simulink model "sampleModel1"  (R2021a)
settings: Solver=VariableStepAuto  StartTime=0.0  StopTime=50  RelTol=1e-3
undefined symbols (not defined in the file): DiscIntNeverNeededParam, magnitude, Newton, Raphson
libraries: simulink x92, pid_lib x10
(part 5 of 5)

== system sampleModel1/cfblk91/cfblk18/cfblk15/cfblk12 ==
  cfblk1 : Inport
  cfblk15 : Inport  Port=2
  cfblk16 : Inport  Port=3
  Action Port : ActionPort  ActionPortLabel=else
  cfblk10 : Constant  Value=[-246777843.934526]  SampleTime=1
  cfblk11 : Constant  Value=[569704854.566047]  SampleTime=1
  cfblk12 : Constant  Value=[627953853.641868]  SampleTime=1
  cfblk13 : Constant  Value=[-141522913.770345]  SampleTime=1
  cfblk14 : Constant  Value=[193294208.890492]  SampleTime=1
  cfblk3 : pid_lib/PID Controller  Controller=PID  Form=Parallel  TimeDomain=Discrete-time  UseExternalTs=off  SampleTime=-1  IntegratorMethod=Forward Euler  FilterMethod=Forward Euler  ControllerParametersSource=internal  P=1  I=1  D=0  UseFilter=on  N=100  TunerSelectOption=Transfer Function Based (PID Tuner App)  InitialConditionSource=internal  InitialConditionForIntegrator=0  InitialConditionForFilter=0  DifferentiatorICPrevScaledInput=0  ExternalReset=none  TrackingMode=off  Kt=1  LimitOutput=off  SatLimitsSource=internal  UpperSaturationLimit=inf  LowerSaturationLimit=-inf  LinearizeAsGain=off  AntiWindupMode=none  Kb=1  POutMin=[]  POutMax=[]  IOutMin=[]  IOutMax=[]  DOutMin=[]  DOutMax=[]  NOutMin=[]  NOutMax=[]  SumOutMin=[]  SumOutMax=[]  SaturationOutMin=[]  SaturationOutMax=[]  PParamMin=[]  PParamMax=[]  IParamMin=[]  IParamMax=[]  DParamMin=[]  DParamMax=[]  NParamMin=[]  NParamMax=[]  KbParamMin=[]  KbParamMax=[]  KtParamMin=[]  KtParamMax=[]  KbOutMin=[]  KbOutMax=[]  KtOutMin=[]  KtOutMax=[]  IntegratorOutMin=[]  IntegratorOutMax=[]  FilterOutMin=[]  FilterOutMax=[]  SumI1OutMin=[]  SumI1OutMax=[]  SumI2OutMin=[]  SumI2OutMax=[]  SumI3OutMin=[]  SumI3OutMax=[]  SumI4OutMin=[]  SumI4OutMax=[]  SumDOutMin=[]  SumDOutMax=[]  DifferentiatorOutMin=[]  DifferentiatorOutMax=[]  FilterDiffOutCoefMin=[]  FilterDiffOutCoefMax=[]  ReciprocalOutMin=[]  ReciprocalOutMax=[]  SumDenOutMin=[]  SumDenOutMax=[]  SumNumOutMin=[]  SumNumOutMax=[]  DivideOutMin=[]  DivideOutMax=[]  UdiffTsProdOutMin=[]  UdiffTsProdOutMax=[]  NTsProdOutMin=[]  NTsProdOutMax=[]  UintegralTsProdOutMin=[]  UintegralTsProdOutMax=[]  UngainTsProdOutMin=[]  UngainTsProdOutMax=[]  IntegratorContinuousStateAttributes=''  IntegratorStateMustResolveToSignalObject=off  IntegratorRTWStateStorageClass=Auto  FilterContinuousStateAttributes=''  FilterStateMustResolveToSignalObject=off  FilterRTWStateStorageClass=Auto  ParallelPVariant=InternalParameters  IdealPVariant=Disabled  IVariant=InternalParameters  DVariant=InternalParameters  IntegratorVariant=Discrete  SatVariant=Disabled  AWVariant=Passthrough  PCopyVariant=Disabled  TRVariant=Disabled  FdbkBlocksVariant=Forward  IdealPFdbkVariant=Disabled  SatFdbkVariant=Disabled  DerivativeFilterVariant=ForwardEulerFilter  NVariant=InternalParameters  NCopyVariant=Disabled  FilterICVariant=InternalICsFilter  IntegratorICVariant=InternalICs  ExternalResetVariant=Disabled  TRSumVariant=Passthrough  SumFdbkVariant=Disabled  SumVariant=Sum_PID  TsampFilterVariant=InternalTs  TsampNgainVariant=Passthrough  TsampIntegralVariant=Passthrough  ExternalSaturationOutDataTypeStr=Inherit: Same as second input
  cfblk4 : DiscreteZeroPole  Poles=[0 0.5]  Gain=1  SampleTime=-1
  cfblk5 : Gain  Gain=[-57796269.968503]
  cfblk6 : Product  Inputs=**
  cfblk7 : Product  Inputs=**
  cfblk8 : Sum  Inputs=|++
  cfblk9 : Constant  Value=[688974792.966896]  SampleTime=1
  cfblk2 : Outport
  cfblk17 : Outport  Port=2
  wires:
  cfblk8/1 -> cfblk7/1
  cfblk16/1 -> cfblk7/2
  cfblk10/1 -> cfblk5/1
  cfblk1/1 -> cfblk3/1
  cfblk4/1 -> cfblk2/1
  cfblk3/1 -> cfblk6/1
  cfblk12/1 -> cfblk17/1
  cfblk5/1 -> cfblk4/1
  cfblk11/1 -> cfblk6/2
  cfblk6/1 -> cfblk8/1
  cfblk9/1 -> cfblk8/2

== system sampleModel1/cfblk91/cfblk18/cfblk15/cfblk9 ==
  cfblk1 : Inport
  cfblk7 : Inport  Port=2
  Action Port : ActionPort  ActionPortLabel=if(u1 >= 0)
  cfblk3 : DiscreteIntegrator  SampleTime=-1  ICPrevOutput=DiscIntNeverNeededParam  ICPrevScaledInput=DiscIntNeverNeededParam
  cfblk4 : Squeeze
  cfblk5 : Constant  Value=[717518068.143608]  SampleTime=1
  cfblk6 : Constant  Value=[-364333892.547543]  SampleTime=1
  cfblk2 : Outport
  wires:
  cfblk1/1 -> cfblk4/1
  cfblk4/1 -> cfblk2/1
  cfblk7/1 -> cfblk3/1

== system sampleModel1/cfblk92/cfblk17/cfblk11/cfblk14 ==
  cfblk1 : Inport
  cfblk10 : Inport  Port=2
  cfblk11 : Inport  Port=3
  cfblk12 : Inport  Port=4
  cfblk13 : Inport  Port=5
  cfblk14 : Inport  Port=6
  Action Port : ActionPort  ActionPortLabel=if(u1 >= 0)
  cfblk3 : Gain  Gain=[-441921625.450770]
  cfblk4 : PermuteDimensions
  cfblk5 : Sqrt  SaturateOnIntegerOverflow=on
  cfblk6 : simulink/Math Operations/MinMax Running Resettable  Function=min  vinit=0.0
  cfblk7 : PermuteDimensions
  cfblk8 : Constant  Value=[350750636.833189]  SampleTime=1
  cfblk9 : Constant  Value=[817051797.696749]  SampleTime=1
  cfblk2 : Outport
  cfblk15 : Outport  Port=2
  wires:
  cfblk11/1 -> cfblk3/1
  cfblk3/1 -> cfblk2/1
  cfblk5/1 -> cfblk4/1
  cfblk1/1 -> cfblk7/1
  cfblk12/1 -> cfblk15/1
  cfblk9/1 -> cfblk6/1
  cfblk14/1 -> cfblk6/2
  cfblk6/1 -> cfblk5/1

== system sampleModel1/cfblk92/cfblk17/cfblk11/cfblk15 ==
  cfblk1 : Inport
  Action Port : ActionPort  ActionPortLabel=else
  cfblk10 : Trigonometry
  cfblk11 : Constant  Value=[197257053.266469]  SampleTime=1
  cfblk12 : Constant  Value=[592490701.451690]  SampleTime=1
  cfblk13 : Constant  Value=[-859572952.026083]  SampleTime=1
  cfblk14 : Constant  Value=[-727985222.759821]  SampleTime=1
  cfblk18 : Delay
  cfblk19 : Delay
  cfblk3 : DiscreteIntegrator  SampleTime=-1  ICPrevOutput=DiscIntNeverNeededParam  ICPrevScaledInput=DiscIntNeverNeededParam
  cfblk4 : Delay
  cfblk5 : Squeeze
  cfblk6 : Math  SaturateOnIntegerOverflow=on
  cfblk7 : Sum  Inputs=+-
  cfblk8 : DotProduct  InputSameDT=on  OutDataTypeStr=Inherit: Inherit via internal rule
  cfblk9 : Sum  Inputs=+-
  cfblk2 : Outport
  cfblk15 : Outport  Port=2
  cfblk16 : Outport  Port=3
  cfblk17 : Outport  Port=4
  wires:
  cfblk5/1 -> cfblk6/1, cfblk18/1
  cfblk3/1 -> cfblk5/1
  cfblk11/1 -> cfblk16/1
  cfblk9/1 -> cfblk10/1
  cfblk6/1 -> cfblk8/1, cfblk7/2
  cfblk1/1 -> cfblk9/1
  cfblk7/1 -> cfblk4/1
  cfblk14/1 -> cfblk17/1
  cfblk10/1 -> cfblk2/1
  cfblk8/1 -> cfblk9/2
  cfblk12/1 -> cfblk15/1
  cfblk13/1 -> cfblk8/2
  cfblk18/1 -> cfblk3/1
  cfblk4/1 -> cfblk19/1
  cfblk19/1 -> cfblk7/1

== system sampleModel1/cfblk92/cfblk17/cfblk11/cfblk7 ==
  cfblk1 : Inport
  cfblk10 : Constant  Value=[697193350.959098]  SampleTime=1
  cfblk11 : Constant  Value=[-67596332.418728]  SampleTime=1
  cfblk12 : Constant  Value=[260410249.999499]  SampleTime=1
  cfblk3 : DiscreteFilter
  cfblk4 : simulink/Discrete/Difference  ICPrevInput=0.0  OutMin=[]  OutMax=[]  OutDataTypeStr=Inherit: Inherit via back propagation  OutDataType=fixdt(1, 16)  OutScaling=2^-10  DoSatur=off
  cfblk5 : simulink/Math Operations/Slider Gain  gain=1  low=0  high=2
  cfblk6 : Gain  Gain=[566531874.808073]
  cfblk7 : Sum  Inputs=|++
  cfblk8 : simulink/Math Operations/MinMax Running Resettable  Function=min  vinit=0.0
  cfblk9 : Constant  Value=[-772138722.643148]  SampleTime=1
  cfblk2 : Outport
  cfblk13 : Outport  Port=2
  cfblk14 : Outport  Port=3
  wires:
  cfblk9/1 -> cfblk7/1
  cfblk6/1 -> cfblk7/2
  cfblk7/1 -> cfblk2/1
  cfblk1/1 -> cfblk5/1
  cfblk8/1 -> cfblk6/1
  cfblk11/1 -> cfblk8/1
  cfblk12/1 -> cfblk13/1
  cfblk4/1 -> cfblk3/1
  cfblk10/1 -> cfblk8/2
  cfblk3/1 -> cfblk14/1
  cfblk5/1 -> cfblk4/1

== system sampleModel1/cfblk92/cfblk17/cfblk11/cfblk8 ==
  cfblk1 : Inport
  cfblk12 : Inport  Port=2
  cfblk13 : Inport  Port=3
  cfblk14 : Inport  Port=4
  cfblk10 : Constant  Value=[633710347.547700]  SampleTime=1
  cfblk11 : Constant  Value=[388701121.244883]  SampleTime=1
  cfblk3 : simulink/Discrete/Difference  ICPrevInput=0.0  OutMin=[]  OutMax=[]  OutDataTypeStr=Inherit: Inherit via back propagation  OutDataType=fixdt(1, 16)  OutScaling=2^-10  DoSatur=off
  cfblk4 : Sum  Inputs=|++
  cfblk5 : Abs
  cfblk6 : Gain  Gain=[852588536.395900]
  cfblk7 : Constant  Value=[-863639126.345931]  SampleTime=1
  cfblk8 : Constant  Value=[274302445.050449]  SampleTime=1
  cfblk9 : Constant  Value=[729244025.067106]  SampleTime=1
  cfblk2 : Outport
  cfblk15 : Outport  Port=2
  wires:
  cfblk11/1 -> cfblk5/1
  cfblk7/1 -> cfblk15/1
  cfblk1/1 -> cfblk2/1
  cfblk13/1 -> cfblk4/1
  cfblk5/1 -> cfblk6/1
  cfblk9/1 -> cfblk4/2
  cfblk4/1 -> cfblk3/1

== system sampleModel1/cfblk92/cfblk18/cfblk10/cfblk11 ==
  cfblk1 : Inport
  cfblk6 : Inport  Port=2
  cfblk7 : Inport  Port=3
  cfblk3 : DiscreteFilter
  cfblk4 : Reshape
  cfblk5 : Constant  Value=[-313988376.059350]  SampleTime=1
  cfblk2 : Outport
  cfblk8 : Outport  Port=2
  wires:
  cfblk6/1 -> cfblk8/1
  cfblk4/1 -> cfblk2/1
  cfblk1/1 -> cfblk3/1
  cfblk5/1 -> cfblk4/1

== system sampleModel1/cfblk92/cfblk18/cfblk6/cfblk11 ==
  cfblk1 : Inport
  cfblk11 : Inport  Port=2
  Action Port : ActionPort  ActionPortLabel=if(u1 >= 0)
  cfblk10 : Constant  Value=[-988693863.746309]  SampleTime=1
  cfblk3 : simulink/Math Operations/MinMax Running Resettable  Function=min  vinit=0.0
  cfblk4 : Product  Inputs=**
  cfblk5 : Product  Inputs=**
  cfblk6 : Product
  cfblk7 : Constant  Value=[-726696956.202840]  SampleTime=1
  cfblk8 : Constant  Value=[-600331750.665850]  SampleTime=1
  cfblk9 : Constant  Value=[86089967.308776]  SampleTime=1
  cfblk2 : Outport
  cfblk12 : Outport  Port=2
  wires:
  cfblk5/1 -> cfblk6/1
  cfblk8/1 -> cfblk2/1
  cfblk10/1 -> cfblk3/1, cfblk4/2
  cfblk3/1 -> cfblk5/1
  cfblk9/1 -> cfblk12/1
  cfblk1/1 -> cfblk6/2
  cfblk7/1 -> cfblk3/2
  cfblk11/1 -> cfblk5/2
  cfblk6/1 -> cfblk4/1

== system sampleModel1/cfblk92/cfblk18/cfblk6/cfblk12 ==
  cfblk1 : Inport
  cfblk10 : Inport  Port=2
  cfblk11 : Inport  Port=3
  Action Port : ActionPort  ActionPortLabel=else
  cfblk3 : simulink/Discrete/Difference  ICPrevInput=0.0  OutMin=[]  OutMax=[]  OutDataTypeStr=Inherit: Inherit via back propagation  OutDataType=fixdt(1, 16)  OutScaling=2^-10  DoSatur=off
  cfblk4 : DiscreteFir
  cfblk5 : Abs
  cfblk6 : simulink/Math Operations/MinMax Running Resettable  Function=min  vinit=0.0
  cfblk7 : Constant  Value=[82707866.615409]  SampleTime=1
  cfblk8 : Constant  Value=[-403001105.881521]  SampleTime=1
  cfblk9 : Constant  Value=[718960214.413579]  SampleTime=1
  cfblk2 : Outport
  cfblk12 : Outport  Port=2
  cfblk13 : Outport  Port=3
  cfblk14 : Outport  Port=4
  wires:
  cfblk7/1 -> cfblk3/1
  cfblk5/1 -> cfblk13/1
  cfblk9/1 -> cfblk12/1
  cfblk6/1 -> cfblk5/1
  cfblk1/1 -> cfblk14/1
  cfblk8/1 -> cfblk2/1
  cfblk11/1 -> cfblk6/1
  cfblk3/1 -> cfblk4/1
  cfblk4/1 -> cfblk6/2

== system sampleModel1/cfblk96/cfblk11/cfblk11/cfblk13 ==
  cfblk1 : Inport
  cfblk10 : Inport  Port=2
  cfblk11 : Inport  Port=3
  cfblk3 : Reshape
  cfblk4 : Bias  Bias=[963192417.832765]
  cfblk5 : MinMax
  cfblk6 : Assignment  DiagnosticForDimensions=Warning  IndexOptions=Index vector (dialog)  Indices=1  OutputSizes=1
  cfblk7 : Sin  TimeSource=Use external signal  SampleTime=0
  cfblk8 : Constant  Value=[-892336902.060979]  SampleTime=1
  cfblk9 : Constant  Value=[786948623.480371]  SampleTime=1
  cfblk2 : Outport
  cfblk12 : Outport  Port=2
  wires:
  cfblk7/1 -> cfblk5/1
  cfblk11/1 -> cfblk2/1
  cfblk3/1 -> cfblk4/1
  cfblk6/1 -> cfblk7/1
  cfblk8/1 -> cfblk6/1
  cfblk9/1 -> cfblk12/1
  cfblk1/1 -> cfblk3/1
  cfblk4/1 -> cfblk6/2

== system sampleModel1/cfblk96/cfblk11/cfblk11/cfblk16 ==
  cfblk1 : Inport
  cfblk13 : Inport  Port=2
  Action Port : ActionPort  ActionPortLabel=if(u1 >= 0)
  cfblk10 : Constant  Value=[505715682.206019]  SampleTime=1
  cfblk11 : Constant  Value=[194090459.228806]  SampleTime=1
  cfblk12 : Constant  Value=[461436034.643181]  SampleTime=1
  cfblk3 : Delay
  cfblk4 : Sin  TimeSource=Use external signal  SampleTime=0
  cfblk5 : Sum  Inputs=--
  cfblk6 : UnaryMinus
  cfblk7 : Constant  Value=[26727972.315309]  SampleTime=1
  cfblk8 : Constant  Value=[-480069442.566265]  SampleTime=1
  cfblk9 : Constant  Value=[986685527.683017]  SampleTime=1
  cfblk2 : Outport
  wires:
  cfblk7/1 -> cfblk2/1
  cfblk3/1 -> cfblk5/1
  cfblk10/1 -> cfblk4/1
  cfblk5/1 -> cfblk6/1
  cfblk13/1 -> cfblk3/1
  cfblk4/1 -> cfblk5/2

== system sampleModel1/cfblk96/cfblk11/cfblk11/cfblk17 ==
  cfblk1 : Inport
  cfblk14 : Inport  Port=2
  Action Port : ActionPort  ActionPortLabel=else
  cfblk10 : Sin  TimeSource=Use external signal  SampleTime=0
  cfblk11 : Constant  Value=[157144619.707222]  SampleTime=1
  cfblk12 : Constant  Value=[791193052.288790]  SampleTime=1
  cfblk13 : Constant  Value=[-114520044.472529]  SampleTime=1
  cfblk3 : DiscreteStateSpace  SampleTime=-1
  cfblk4 : Rounding
  cfblk5 : ComplexToRealImag
  cfblk6 : ComplexToRealImag
  cfblk7 : Sum  Inputs=|++
  cfblk8 : Sum  Inputs=-+
  cfblk9 : UnaryMinus
  cfblk2 : Outport
  cfblk15 : Outport  Port=2
  wires:
  cfblk11/1 -> cfblk2/1
  cfblk6/1 -> cfblk4/1
  cfblk13/1 -> cfblk7/1
  cfblk12/1 -> cfblk3/1
  cfblk4/1 -> cfblk7/2
  cfblk9/1 -> cfblk8/1
  cfblk3/1 -> cfblk6/1
  cfblk8/1 -> cfblk15/1
  cfblk14/1 -> cfblk8/2
  cfblk1/1 -> cfblk10/1
  cfblk10/1 -> cfblk5/1
  cfblk5/1 -> cfblk9/1

== system sampleModel1/cfblk99/cfblk9/cfblk12/cfblk16 ==
  cfblk1 : Inport
  cfblk11 : Inport  Port=2
  Action Port : ActionPort  ActionPortLabel=if(u1 >= 0)
  cfblk10 : Constant  Value=[905056290.746794]  SampleTime=1
  cfblk3 : simulink/Discrete/Difference  ICPrevInput=0.0  OutMin=[]  OutMax=[]  OutDataTypeStr=Inherit: Inherit via back propagation  OutDataType=fixdt(1, 16)  OutScaling=2^-10  DoSatur=off
  cfblk4 : DotProduct  InputSameDT=on  OutDataTypeStr=Inherit: Inherit via internal rule
  cfblk5 : Product  Inputs=*
  cfblk6 : simulink/Math Operations/Slider Gain  gain=1  low=0  high=2
  cfblk7 : Constant  Value=[-82052266.355280]  SampleTime=1
  cfblk8 : Constant  Value=[321672188.896489]  SampleTime=1
  cfblk9 : Constant  Value=[-305627404.212235]  SampleTime=1
  cfblk2 : Outport
  cfblk12 : Outport  Port=2
  wires:
  cfblk5/1 -> cfblk2/1
  cfblk9/1 -> cfblk6/1
  cfblk1/1 -> cfblk5/1
  cfblk11/1 -> cfblk4/1
  cfblk7/1 -> cfblk3/1
  cfblk3/1 -> cfblk4/2
  cfblk10/1 -> cfblk12/1

== system sampleModel1/cfblk99/cfblk9/cfblk12/cfblk17 ==
  cfblk1 : Inport
  cfblk10 : Inport  Port=2
  cfblk11 : Inport  Port=3
  cfblk12 : Inport  Port=4
  cfblk13 : Inport  Port=5
  cfblk14 : Inport  Port=6
  cfblk15 : Inport  Port=7
  Action Port : ActionPort  ActionPortLabel=else
  cfblk18 : Delay
  cfblk3 : Bias  Bias=[611676517.589504]
  cfblk4 : PermuteDimensions
  cfblk5 : Product
  cfblk6 : Product  Inputs=*
  cfblk7 : Sum  Inputs=+-
  cfblk8 : Signum
  cfblk9 : Constant  Value=[62485738.917163]  SampleTime=1
  cfblk2 : Outport
  cfblk16 : Outport  Port=2
  cfblk17 : Outport  Port=3
  wires:
  cfblk9/1 -> cfblk2/1
  cfblk4/1 -> cfblk8/1
  cfblk6/1 -> cfblk7/1
  cfblk3/1 -> cfblk17/1
  cfblk15/1 -> cfblk3/1
  cfblk5/1 -> cfblk4/1
  cfblk1/1 -> cfblk5/2
  cfblk13/1 -> cfblk7/2
  cfblk12/1 -> cfblk16/1
  cfblk10/1 -> cfblk6/1
  cfblk8/1 -> cfblk18/1
  cfblk18/1 -> cfblk5/1

== system sampleModel1/cfblk99/cfblk9/cfblk13/cfblk11 ==
  cfblk1 : Inport
  cfblk14 : Inport  Port=2
  cfblk15 : Inport  Port=3
  cfblk16 : Inport  Port=4
  cfblk10 : Constant  Value=[562169036.002765]  SampleTime=1
  cfblk11 : Constant  Value=[986686499.861837]  SampleTime=1
  cfblk12 : Constant  Value=[301237087.815454]  SampleTime=1
  cfblk13 : Constant  Value=[-512253795.715361]  SampleTime=1
  cfblk3 : DiscreteFir
  cfblk4 : Product  Inputs=**
  cfblk5 : Polyval  Coefs=[ +2.081618890e-019, -1.441693666e-014, +4.719686976e-010, -8.536869453e-006, +1.621573104e-001, -8.087801117e+001 ]
  cfblk6 : DotProduct  InputSameDT=on  OutDataTypeStr=Inherit: Inherit via internal rule
  cfblk7 : Sum  Inputs=--
  cfblk8 : ComplexToRealImag
  cfblk9 : Constant  Value=[416226752.813493]  SampleTime=1
  cfblk2 : Outport
  cfblk17 : Outport  Port=2
  wires:
  cfblk10/1 -> cfblk3/1
  cfblk7/1 -> cfblk17/1
  cfblk12/1 -> cfblk6/1
  cfblk6/1 -> cfblk7/1
  cfblk16/1 -> cfblk8/1
  cfblk4/1 -> cfblk6/2
  cfblk3/1 -> cfblk7/2
  cfblk11/1 -> cfblk4/1
  cfblk9/1 -> cfblk5/1
  cfblk15/1 -> cfblk4/2
  cfblk1/1 -> cfblk2/1

== system sampleModel1/cfblk99/cfblk9/cfblk13/cfblk12 ==
  cfblk1 : Inport
  cfblk12 : Inport  Port=2
  cfblk10 : Constant  Value=[-78703613.587570]  SampleTime=1
  cfblk11 : Constant  Value=[-830746722.847237]  SampleTime=1
  cfblk3 : Product  Inputs=*
  cfblk4 : Rounding
  cfblk5 : UnaryMinus
  cfblk6 : Signum
  cfblk7 : Gain  Gain=[-997073649.655154]
  cfblk8 : Constant  Value=[767577618.804535]  SampleTime=1
  cfblk9 : Constant  Value=[-397588826.973055]  SampleTime=1
  cfblk2 : Outport
  cfblk13 : Outport  Port=2
  cfblk14 : Outport  Port=3
  cfblk15 : Outport  Port=4
  cfblk16 : Outport  Port=5
  wires:
  cfblk1/1 -> cfblk3/1
  cfblk5/1 -> cfblk13/1
  cfblk10/1 -> cfblk5/1
  cfblk6/1 -> cfblk16/1
  cfblk12/1 -> cfblk15/1
  cfblk9/1 -> cfblk4/1
  cfblk11/1 -> cfblk7/1
  cfblk7/1 -> cfblk6/1
  cfblk4/1 -> cfblk14/1
  cfblk3/1 -> cfblk2/1

== system sampleModel1/cfblk99/cfblk9/cfblk13/cfblk15 ==
  cfblk1 : Inport
  cfblk11 : Inport  Port=2
  Action Port : ActionPort  ActionPortLabel=if(u1 >= 0)
  cfblk10 : Constant  Value=[-585686707.710084]  SampleTime=1
  cfblk3 : Reshape
  cfblk4 : ComplexToMagnitudeAngle
  cfblk5 : Squeeze
  cfblk6 : Rounding
  cfblk7 : Product  Inputs=*
  cfblk8 : Sum
  cfblk9 : Constant  Value=[266910070.024732]  SampleTime=1
  cfblk2 : Outport
  cfblk12 : Outport  Port=2
  cfblk13 : Outport  Port=3
  cfblk14 : Outport  Port=4
  wires:
  cfblk6/1 -> cfblk13/1
  cfblk10/1 -> cfblk3/1
  cfblk1/1 -> cfblk6/1
  cfblk8/1 -> cfblk14/1
  cfblk11/1 -> cfblk2/1
  cfblk3/1 -> cfblk4/1
  cfblk7/1 -> cfblk12/1
  cfblk5/1 -> cfblk7/1
  cfblk4/1 -> cfblk8/1
  cfblk9/1 -> cfblk8/2
  cfblk4/2 -> cfblk5/1

== system sampleModel1/cfblk99/cfblk9/cfblk13/cfblk16 ==
  cfblk1 : Inport
  Action Port : ActionPort  ActionPortLabel=else
  cfblk3 : Squeeze
  cfblk4 : Sum  Inputs=+
  cfblk5 : Sin  TimeSource=Use external signal  SampleTime=0
  cfblk6 : Sum  Inputs=|++
  cfblk7 : Gain  Gain=[849096615.239038]
  cfblk8 : Signum
  cfblk9 : Constant  Value=[-837494449.259007]  SampleTime=1
  cfblk2 : Outport
  cfblk10 : Outport  Port=2
  wires:
  cfblk4/1 -> cfblk3/1
  cfblk3/1 -> cfblk10/1
  cfblk7/1 -> cfblk2/1
  cfblk6/1 -> cfblk5/1
  cfblk9/1 -> cfblk8/1
  cfblk5/1 -> cfblk7/1, cfblk4/1
  cfblk1/1 -> cfblk6/1
  cfblk8/1 -> cfblk6/2
